simulink model "ICC_MRAC"  (Simulink 5.0)
settings: Solver=ode45  StartTime=0.0  StopTime=180  MaxStep=.01  RelTol=1e-3
values from neighbouring files (symbols this model uses):
  am = 1.0    (= 1)    [ICC.m]
  gamma1 = 0.8    [ICC.m]
  gamma2 = 0.3    [ICC.m]
  gamma3 = 0.3    [ICC.m]
  h = 1.0    (= 1)    [ICC.m]
  k = 0.4    [ICC.m]
  k1_0 = 6.0    (= 6)    [ICC.m]
  k1_max = 14.0    (= 14)    [ICC.m]
  k1_min = 4.0    (= 4)    [ICC.m]
  k2_0 = 2.0    (= 2)    [ICC.m]
  k2_max = 4.0    (= 4)    [ICC.m]
  k2_min = 0.5    [ICC.m]
  k3_0 = 0.0    (= 0)    [ICC.m]
  k3_max = 30.0    (= 30)    [ICC.m]
  k3_min = -30.0    (= -30)    [ICC.m]
  lambda = 0.1    [ICC.m]
  s0 = 4.5    [ICC.m]
  v0 = 0    [ICC.m]
undefined symbols (not defined in the file or in its folder): eng_tbl, gearshift, SwitchLogic
libraries: simulink x8, simulink_extras x1
settings Model: LastModifiedBy=Administrator  BlockReductionOpt=off  BooleanDataType=off

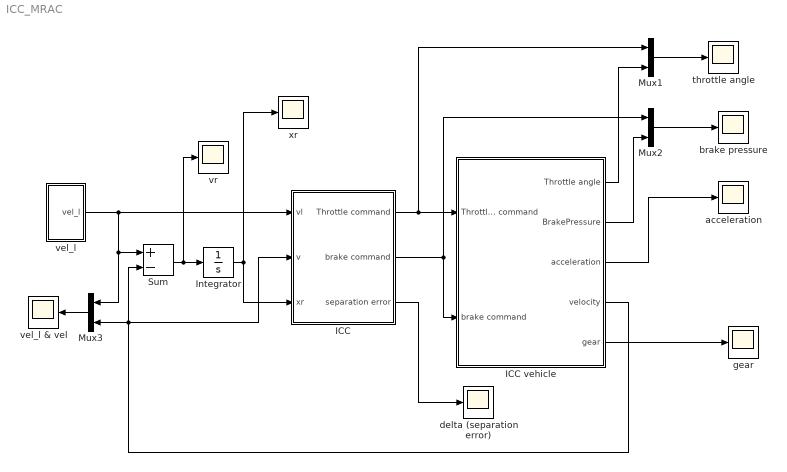
== system ICC_MRAC ==
  ICC : Subsystem
  ICC vehicle : Subsystem
  Integrator : Integrator  InitialCondition=s0
  Mux1 : Mux  Inputs=2
  Mux2 : Mux  Inputs=2
  Mux3 : Mux  Orientation=left  Inputs=2
  Sum : Sum  Inputs=+-  SaturateOnIntegerOverflow=on  InputSameDT=on
  acceleration : Scope
      settings: YMin=-1  YMax=4  SaveName=a  DataFormat=Array  SampleInput=on  SampleTime=0.1
  brake pressure : Scope
      settings: YMin=0  YMax=800  SaveName=brk_pressure  DataFormat=Array  SampleInput=on  SampleTime=0.1
  delta (separation error) : Scope
      settings: YMin=-0.0025  YMax=0.02  SaveName=posit_err  DataFormat=Array  SampleInput=on  SampleTime=0.1
  gear : Scope
      settings: SaveName=gear  DataFormat=Array  SampleInput=on  SampleTime=0.1
  throttle angle : Scope
      settings: YMin=0  YMax=45  SaveName=thrt_angle  DataFormat=Array  SampleInput=on  SampleTime=0.1
  vel_l : Subsystem
  vel_l & vel : Scope
      settings: YMin=0  YMax=30  SaveName=v  DataFormat=Array  SampleInput=on  SampleTime=0.1
  vr : Scope
      settings: YMin=-2  YMax=4  SaveName=vr  DataFormat=Array  SampleInput=on  SampleTime=0.1
  xr : Scope
      settings: YMin=0  YMax=45  SaveName=xr  DataFormat=Array  SampleInput=on  SampleTime=0.1
  wires:
  Sum/1 -> Integrator/1, vr/1
  Integrator/1 -> xr/1, ICC/3(xr)
  Mux1/1 -> throttle angle/1
  Mux2/1 -> brake pressure/1
  vel_l/1(vel_l) -> Sum/1, Mux3/1, ICC/1(vl)
  Mux3/1 -> vel_l & vel/1
  ICC vehicle/4(velocity) -> Mux3/2, Sum/2, ICC/2(v)
  ICC/2(brake command) -> ICC vehicle/2(brake command), Mux2/1
  ICC/1(Throttle command) -> ICC vehicle/1(Throttle command), Mux1/1
  ICC vehicle/1(Throttle angle) -> Mux1/2
  ICC vehicle/2(BrakePressure) -> Mux2/2
  ICC vehicle/3(acceleration) -> acceleration/1
  ICC vehicle/5(gear) -> gear/1
  ICC/3(separation error) -> delta (separation error)/1

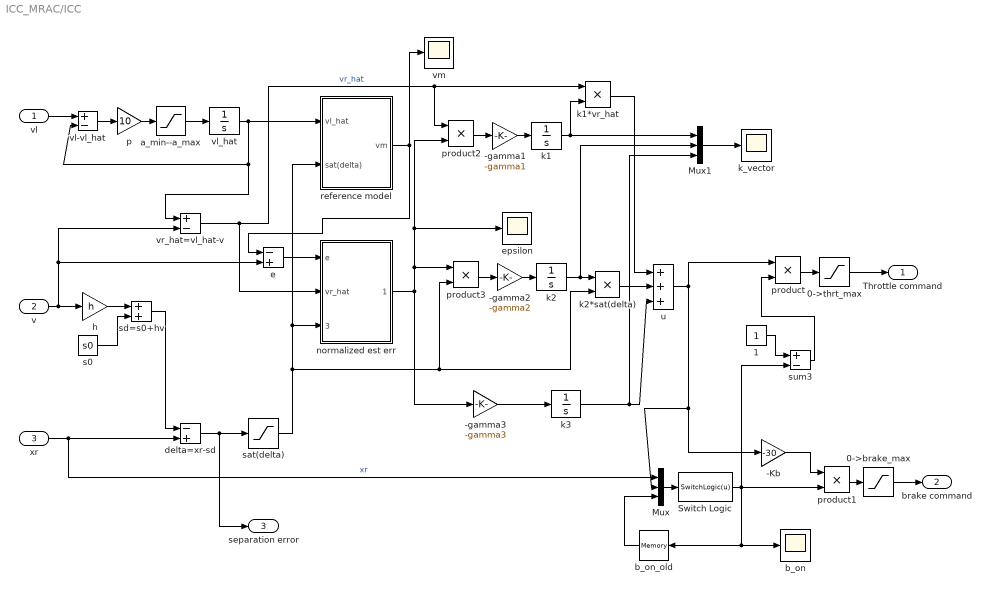
== system ICC_MRAC/ICC ==
  vl : Inport
  v : Inport  Port=2
  xr : Inport  Port=3
  -Kb : Gain  Gain=-30  SaturateOnIntegerOverflow=on
  -gamma1 : Gain  Gain=-gamma1  SaturateOnIntegerOverflow=on
  -gamma2 : Gain  Gain=-gamma2  SaturateOnIntegerOverflow=on
  -gamma3 : Gain  Gain=-gamma3  SaturateOnIntegerOverflow=on
  0->brake_max : Saturate  UpperLimit=800  LowerLimit=0
  0->thrt_max : Saturate  UpperLimit=85  LowerLimit=0
  1 : Constant
  Mux : Mux  Inputs=3
  Mux1 : Mux  Inputs=3
  Switch Logic : MATLABFcn  MATLABFcn=SwitchLogic(u)
  a_min--a_max : Saturate  UpperLimit=1.0  LowerLimit=-2.0
  b_on : Scope
      settings: YMin=-1  YMax=1  SaveName=b_on  DataFormat=Array  SampleInput=on  SampleTime=0.1
  b_on_old : Memory  Orientation=left
  delta=xr-sd : Sum  Inputs=-+  SaturateOnIntegerOverflow=on  InputSameDT=on
  e : Sum  Inputs=-+  SaturateOnIntegerOverflow=on  InputSameDT=on
  epsilon : Scope
      settings: YMin=4  YMax=9.5  SaveName=epsilon  DataFormat=Array  SampleInput=on  SampleTime=0.1
  h : Gain  Gain=h  SaturateOnIntegerOverflow=on
  k1 : Integrator  InitialCondition=k1_0  LimitOutput=on  UpperSaturationLimit=k1_max  LowerSaturationLimit=k1_min
  k1*vr_hat : Product  SaturateOnIntegerOverflow=on  InputSameDT=on
  k2 : Integrator  InitialCondition=k2_0  LimitOutput=on  UpperSaturationLimit=k2_max  LowerSaturationLimit=k2_min
  k2*sat(delta) : Product  SaturateOnIntegerOverflow=on  InputSameDT=on
  k3 : Integrator  InitialCondition=k3_0  LimitOutput=on  UpperSaturationLimit=k3_max  LowerSaturationLimit=k3_min
  k_vector : Scope
      settings: YMin=4  YMax=9.5  SaveName=k_vector  DataFormat=Array  SampleInput=on  SampleTime=0.1
  normalized est err : Subsystem
  p : Gain  Gain=10  SaturateOnIntegerOverflow=on
  product{,1..3} (4 alike) : Product  SaturateOnIntegerOverflow=on  InputSameDT=on
  reference model : Subsystem
  s0 : Constant  Value=s0
  sat(delta) : Saturate  UpperLimit=5  LowerLimit=-10
  sd=s0+hv : Sum  SaturateOnIntegerOverflow=on  InputSameDT=on
  sum3 : Sum  Inputs=+-  SaturateOnIntegerOverflow=on  InputSameDT=on
  u : Sum  Inputs=+++  SaturateOnIntegerOverflow=on  InputSameDT=on
  vl-vl_hat : Sum  Inputs=+-  SaturateOnIntegerOverflow=on  InputSameDT=on
  vl_hat : Integrator  InitialCondition=v0
  vm : Scope
      settings: YMin=4  YMax=9.5  SaveName=vm  DataFormat=Array  SampleInput=on  SampleTime=0.1
  vr_hat=vl_hat-v : Sum  Inputs=+-  SaturateOnIntegerOverflow=on  InputSameDT=on
  Throttle command : Outport  InitialOutput=0
  brake command : Outport  Port=2  InitialOutput=0
  separation error : Outport  Port=3  InitialOutput=0
  wires:
  vl/1 -> vl-vl_hat/1
  a_min--a_max/1 -> vl_hat/1
  v/1 -> h/1, vr_hat=vl_hat-v/2, e/2
  s0/1 -> sd=s0+hv/2
  h/1 -> sd=s0+hv/1
  xr/1 -> delta=xr-sd/2, Mux/1  "xr"
  sd=s0+hv/1 -> delta=xr-sd/1
  vr_hat=vl_hat-v/1 -> normalized est err/2(vr_hat), product2/1, k1*vr_hat/1  "vr_hat"
  delta=xr-sd/1 -> separation error/1, sat(delta)/1
  sat(delta)/1 -> normalized est err/3(sat(delta)), reference model/2(sat(delta)), k2*sat(delta)/2, product3/2
  k1/1 -> k1*vr_hat/2, Mux1/1
  k2/1 -> k2*sat(delta)/1, Mux1/2
  k3/1 -> u/3, Mux1/3
  k2*sat(delta)/1 -> u/2
  k1*vr_hat/1 -> u/1
  u/1 -> product/1, Mux/2, -Kb/1
  Mux/1 -> Switch Logic/1
  b_on_old/1 -> Mux/3
  1/1 -> sum3/1
  Switch Logic/1 -> sum3/2, product1/2, b_on_old/1, b_on/1
  sum3/1 -> product/2
  product/1 -> 0->thrt_max/1
  0->thrt_max/1 -> Throttle command/1
  -Kb/1 -> product1/1
  product1/1 -> 0->brake_max/1
  0->brake_max/1 -> brake command/1
  Mux1/1 -> k_vector/1
  vl-vl_hat/1 -> p/1
  p/1 -> a_min--a_max/1
  vl_hat/1 -> vl-vl_hat/2, vr_hat=vl_hat-v/1, reference model/1(vl_hat)
  reference model/1(vm) -> vm/1, e/1
  -gamma1/1 -> k1/1
  product2/1 -> -gamma1/1
  normalized est err/1(epsilon) -> product3/1, product2/2, epsilon/1, -gamma3/1
  -gamma2/1 -> k2/1
  product3/1 -> -gamma2/1
  -gamma3/1 -> k3/1
  e/1 -> normalized est err/1(e)

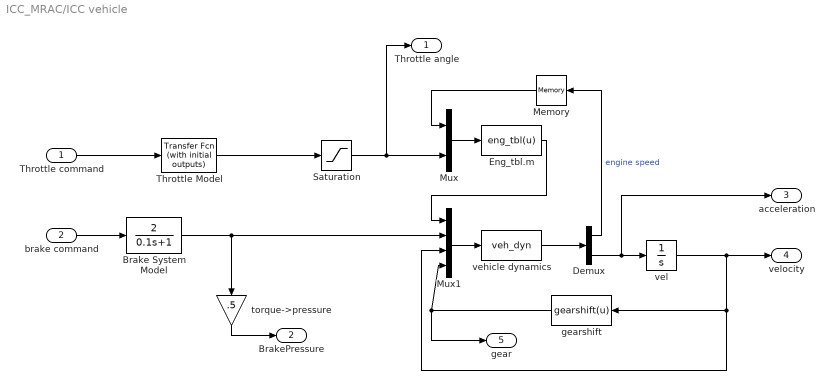
== system ICC_MRAC/ICC vehicle ==
  Throttle command : Inport
  brake command : Inport  Port=2
  Brake System Model : TransferFcn  Numerator=[2]  Denominator=[0.1 1]
  Demux : Demux  Outputs=2
  Eng_tbl.m : MATLABFcn  MATLABFcn=eng_tbl(u)  OutputDimensions=1
  Memory : Memory  Orientation=left
  Mux : Mux  Inputs=2
  Mux1 : Mux
  Saturation : Saturate  UpperLimit=85  LowerLimit=0
  Throttle Model : simulink_extras/Additional Linear/Transfer Fcn (with initial outputs)  N=[1]  D=[0.1 1]  Y0=thrt_init  U0=thrt_init
  gearshift : MATLABFcn  Orientation=left  MATLABFcn=gearshift(u)  OutputDimensions=1
  torque->pressure : Gain  Orientation=down  Gain=.5  SaturateOnIntegerOverflow=on
  vehicle dynamics : MATLABFcn  MATLABFcn=veh_dyn  OutputDimensions=2
  vel : Integrator  InitialCondition=v0  LimitOutput=on  LowerSaturationLimit=0
  Throttle angle : Outport  InitialOutput=0
  BrakePressure : Outport  Port=2  InitialOutput=0
  acceleration : Outport  Port=3  InitialOutput=0
  velocity : Outport  Port=4  InitialOutput=0
  gear : Outport  Port=5  InitialOutput=0
  wires:
  Throttle Model/1 -> Saturation/1
  Brake System Model/1 -> Mux1/2, torque->pressure/1
  Mux/1 -> Eng_tbl.m/1
  Throttle command/1 -> Throttle Model/1
  brake command/1 -> Brake System Model/1
  Demux/1 -> Memory/1  "engine speed"
  vehicle dynamics/1 -> Demux/1
  Mux1/1 -> vehicle dynamics/1
  Eng_tbl.m/1 -> Mux1/1
  vel/1 -> velocity/1, gearshift/1, Mux1/3
  torque->pressure/1 -> BrakePressure/1
  Memory/1 -> Mux/1
  gearshift/1 -> gear/1, Mux1/4
  Saturation/1 -> Throttle angle/1, Mux/2
  Demux/2 -> vel/1, acceleration/1

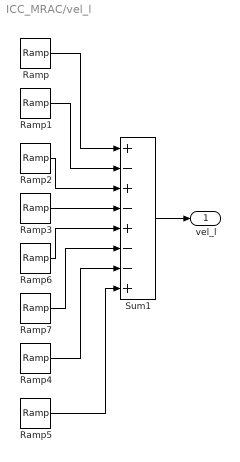
== system ICC_MRAC/vel_l ==
  Ramp : simulink/Sources/Ramp  slope=0.8  start=0  X0=v0
  Ramp1 : simulink/Sources/Ramp  slope=0.8  start=20  X0=0
  Ramp2 : simulink/Sources/Ramp  slope=2  start=50  X0=0
  Ramp3 : simulink/Sources/Ramp  slope=2  start=53  X0=0
  Ramp4 : simulink/Sources/Ramp  slope=2  start=140  X0=0
  Ramp5 : simulink/Sources/Ramp  slope=2  start=144  X0=0
  Ramp6 : simulink/Sources/Ramp  slope=0.6  start=90  X0=0
  Ramp7 : simulink/Sources/Ramp  slope=0.6  start=100  X0=0
  Sum1 : Sum  Inputs=+-+-+--+  SaturateOnIntegerOverflow=on  InputSameDT=on
  vel_l : Outport
  wires:
  Ramp/1 -> Sum1/1
  Ramp1/1 -> Sum1/2
  Ramp2/1 -> Sum1/3
  Ramp3/1 -> Sum1/4
  Sum1/1 -> vel_l/1
  Ramp6/1 -> Sum1/5
  Ramp7/1 -> Sum1/6
  Ramp4/1 -> Sum1/7
  Ramp5/1 -> Sum1/8

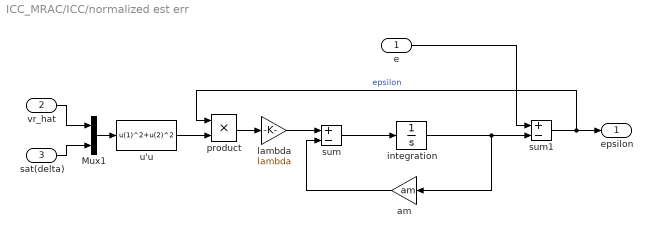
== system ICC_MRAC/ICC/normalized est err ==
  e : Inport
  vr_hat : Inport  Port=2
  sat(delta) : Inport  Port=3
  Mux1 : Mux  Inputs=2
  am : Gain  Orientation=left  Gain=am  SaturateOnIntegerOverflow=on
  integration : Integrator  InitialCondition=v0
  lambda : Gain  Gain=lambda  SaturateOnIntegerOverflow=on
  product : Product  SaturateOnIntegerOverflow=on  InputSameDT=on
  sum : Sum  Inputs=+-  SaturateOnIntegerOverflow=on  InputSameDT=on
  sum1 : Sum  Inputs=+-  SaturateOnIntegerOverflow=on  InputSameDT=on
  u'u : Fcn  Expr=u(1)^2+u(2)^2
  epsilon : Outport  InitialOutput=0
  wires:
  sum/1 -> integration/1
  integration/1 -> am/1, sum1/2
  vr_hat/1 -> Mux1/1
  sat(delta)/1 -> Mux1/2
  Mux1/1 -> u'u/1
  u'u/1 -> product/2
  sum1/1 -> epsilon/1, product/1  "epsilon"
  product/1 -> lambda/1
  am/1 -> sum/2
  e/1 -> sum1/1
  lambda/1 -> sum/1

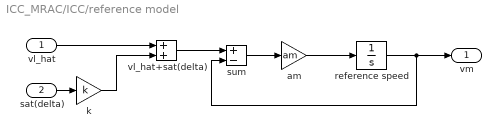
== system ICC_MRAC/ICC/reference model ==
  vl_hat : Inport
  sat(delta) : Inport  Port=2
  am : Gain  Gain=am  SaturateOnIntegerOverflow=on
  k : Gain  Gain=k  SaturateOnIntegerOverflow=on
  reference speed : Integrator  InitialCondition=v0
  sum : Sum  Inputs=+-  SaturateOnIntegerOverflow=on  InputSameDT=on
  vl_hat+sat(delta) : Sum  SaturateOnIntegerOverflow=on  InputSameDT=on
  vm : Outport  InitialOutput=0
  wires:
  sat(delta)/1 -> k/1
  vl_hat/1 -> vl_hat+sat(delta)/1
  k/1 -> vl_hat+sat(delta)/2
  vl_hat+sat(delta)/1 -> sum/1
  sum/1 -> am/1
  reference speed/1 -> vm/1, sum/2
  am/1 -> reference speed/1
